simulink model "Single Phase SPWM"  (R2017a)
settings: Solver=ode23tb  StartTime=0.0  StopTime=0.1  MaxStep=5e-6  RelTol=1e-3  EnableMultiTasking=on
libraries: powerlib x10, simulink x1, powerlib_extras x1
settings Model: Creator=lenova  LastModifiedBy=sujee
settings DataIOCC: LimitDataPoints=on  SaveFormat=Array  SignalLoggingSaveFormat=ModelDataLogs
settings OptimizationCC: ExpressionDepthLimit=2147483647  LifeSpan=inf
settings DebuggingCC: UnderspecifiedInitializationDetection=Classic  MergeDetectMultiDrivingBlocksExec=none  SolverPrmCheckMsg=warning  FcnCallInpInsideContextMsg=warning  StateNameClashWarn=warning  SFUnexpectedBacktrackingDiag=warning  SFNoUnconditionalDefaultTransitionDiag=warning  SFExecutionAtInitializationDiag=none
settings HardwareCC: ProdBitPerPointer=32  ProdBitPerSizeT=32  ProdBitPerPtrDiffT=32  ProdLargestAtomicFloat=None  ProdIntDivRoundTo=Undefined  ProdEndianess=Unspecified  ProdWordSize=32  ProdHWDeviceType=32-bit Generic
settings ModelReferenceCC: PropagateSignalLabelsOutOfModel=off
settings GRTTargetCC: TargetLangStandard=C89/C90 (ANSI)  CombineOutputUpdateFcns=off  GRTInterface=on
settings ConfigComp: CovMetricSettings=dw  CovSaveCumulativeToWorkspaceVar=on  CovSaveSingleToWorkspaceVar=on  CovExternalEMLEnable=off
settings SimscapeCC: SimscapeNormalizeSystem=off

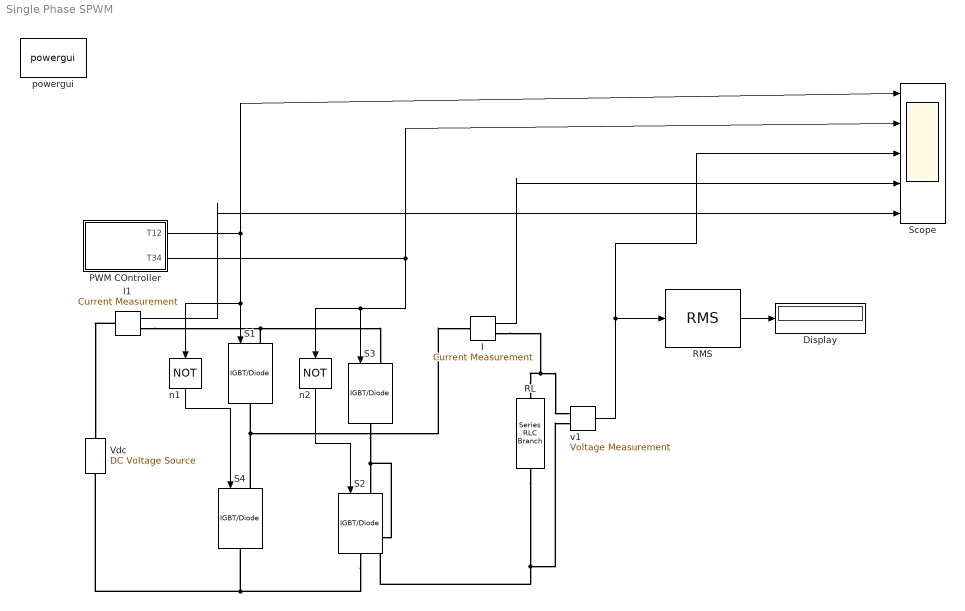
== system Single Phase SPWM ==
  Display : Display
  I : powerlib/Measurements/Current Measurement  PhasorSimulation=off  OutputType=Complex  PSBequivalent=0
  I1 : powerlib/Measurements/Current Measurement  PhasorSimulation=off  OutputType=Complex  PSBequivalent=0
  PWM COntroller : Subsystem  mask{f=50, m=0.7, s=2000}
      mask prompts: f "Output frequency in Ha"; m "Modulation index in pu"; s "Switching frequency in Hz"
  RL : powerlib/Elements/Series RLC Branch  LConnTagsString=__new0  RConnTagsString=__new0  BranchType=RL  Resistance=10  Inductance=10e-3  SetiL0=off  InitialCurrent=0  Capacitance=1e-6  Setx0=off  InitialVoltage=0  Measurements=None
  RMS : powerlib_extras/Measurements/RMS  f1=50
      settings: SourceProductBaseCode=PS
  S{1..4} (4 alike) : powerlib/Power Electronics/IGBT//Diode  Ron=1e-3  Rs=1e5  Cs=inf  Measurements=off
  Scope : Scope  NumInputPorts=5
  Vdc : powerlib/Electrical Sources/DC Voltage Source  Amplitude=325  Measurements=None
  n1 : Logic  Operator=NOT  AllPortsSameDT=off  OutDataTypeStr=boolean
  n2 : Logic  Operator=NOT  AllPortsSameDT=off  OutDataTypeStr=boolean
  powergui : powerlib/powergui  Priority=1  SimulationMode=Continuous  SampleTime=50e-6  frequency=60  Iterations=50  frequencyindice=0  Pbase=100e6  ErrMax=1e-4  UnitsV=kV  UnitsW=MW  buscounter=0  FunctionMessages=off  echomessages=off  EnableUseOfTLC=off  CurrentSourceSwitches=off  DisableSnubberDevices=off  DisableRonSwitches=off  DisableVfSwitches=off  DisplayEquations=off  AutomaticDiscreteSolvers=off  SolverType=Tustin/Backward Euler (TBE)  Interpol=off  ExternalGateDelay=off  methode=off  Ts=10  x0status=blocks  SPID=off  SwTol=0  HookPort=off  NonlinearTolerance=1e-4  nMaxIteration=100  ContinueOnMaxIteration=off  RestoreLinks=warning  ResistiveCurrentMeasurement=off  Frange=[0:2:500]  Ylog=off  Xlog=on  ShowGrid=off  save=off  variable=ZData  structure=0  ZoomFFT=off  StartTime=0.0  cycles=1  DisplayStyle=1  fundamental=60  FreqAxis=off  MaxFrequency=1000  frequencyindicesteady=1  RmsSteady=1  display=off
  v1 : powerlib/Measurements/Voltage Measurement  PhasorSimulation=off  OutputType=Complex  PSBequivalent=0
  wires:
  v1/1 -> RMS/1, Scope/3
  RMS/1 -> Display/1
  I/1 -> Scope/4
  PWM COntroller/1(T12) -> Scope/1, S1/1, n1/1
  PWM COntroller/2(T34) -> Scope/2, S3/1, n2/1
  n1/1 -> S4/1
  n2/1 -> S2/1
  I1/1 -> Scope/5
  connections:
  S1/LConn1 -- S3/LConn1 -- I1/RConn1
  RL/LConn1 -- v1/LConn1 -- I/RConn1
  RL/RConn1 -- v1/LConn2 -- S3/RConn1 -- S2/LConn1
  S2/RConn1 -- S4/RConn1 -- Vdc/LConn1
  S4/LConn1 -- S1/RConn1 -- I/LConn1
  I1/LConn1 -- Vdc/RConn1

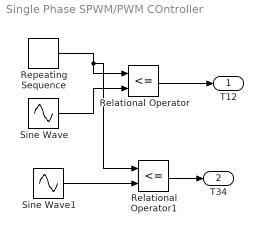
== system Single Phase SPWM/PWM COntroller ==
  Relational Operator : RelationalOperator  Operator=<=  OutDataTypeStr=boolean  RndMeth=Nearest
  Relational Operator1 : RelationalOperator  Operator=<=  OutDataTypeStr=boolean  RndMeth=Nearest
  Repeating Sequence : simulink/Sources/Repeating Sequence  rep_seq_t=[0 1/s]  rep_seq_y=[0 1]
  Sine Wave : Sin  Amplitude=m  Frequency=2*pi*f  SampleTime=0
  Sine Wave1 : Sin  Amplitude=m  Frequency=2*pi*f  Phase=-pi  SampleTime=0
  T12 : Outport
  T34 : Outport  Port=2
  wires:
  Relational Operator/1 -> T12/1
  Relational Operator1/1 -> T34/1
  Repeating Sequence/1 -> Relational Operator/1, Relational Operator1/1
  Sine Wave/1 -> Relational Operator/2
  Sine Wave1/1 -> Relational Operator1/2
